simulink model "aula8_sim"  (R2013b)
settings: Solver=ode45  StartTime=0.0  StopTime=10  RelTol=1e-3
values from neighbouring files (symbols this model uses):
  K = lqr(A,B,Q,R)    [Aula8.m]
settings Model: Creator=ThiagoCordeiro  LastModifiedBy=ThiagoFelippe

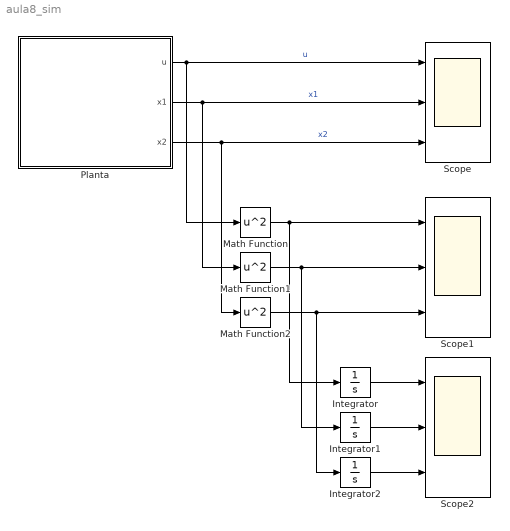
== system aula8_sim ==
  Integrator : Integrator
  Integrator1 : Integrator
  Integrator2 : Integrator
  Math Function : Math  Operator=square  SaturateOnIntegerOverflow=on
  Math Function1 : Math  Operator=square  SaturateOnIntegerOverflow=on
  Math Function2 : Math  Operator=square  SaturateOnIntegerOverflow=on
  Planta : Subsystem
  Scope : Scope  NumInputPorts=3
      settings: ShowLegends=on  YMin=-5~-5~-5  YMax=5~5~5
  Scope1 : Scope  NumInputPorts=3
      settings: YMin=-5~-5~-5  YMax=5~5~5
  Scope2 : Scope  NumInputPorts=3
      settings: YMin=-5~-5~-5  YMax=5~5~5  SaveName=ScopeData2
  wires:
  Planta/1(u) -> Math Function/1, Scope/1  "u"
  Planta/2(x1) -> Math Function1/1, Scope/2  "x1"
  Planta/3(x2) -> Math Function2/1, Scope/3  "x2"
  Math Function/1 -> Integrator/1, Scope1/1
  Math Function2/1 -> Integrator2/1, Scope1/3
  Math Function1/1 -> Integrator1/1, Scope1/2
  Integrator/1 -> Scope2/1
  Integrator1/1 -> Scope2/2
  Integrator2/1 -> Scope2/3

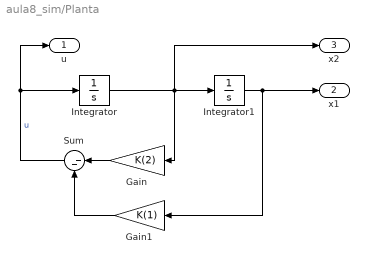
== system aula8_sim/Planta ==
  Gain : Gain  Gain=K(2)
  Gain1 : Gain  Gain=K(1)
  Integrator : Integrator  InitialCondition=5
  Integrator1 : Integrator  InitialCondition=5
  Sum : Sum  Inputs=|--
  u : Outport
  x1 : Outport  Port=2
  x2 : Outport  Port=3
  wires:
  Integrator/1 -> x2/1, Gain/1, Integrator1/1
  Integrator1/1 -> x1/1, Gain1/1
  Sum/1 -> u/1, Integrator/1  "u"
  Gain/1 -> Sum/1
  Gain1/1 -> Sum/2
